simulink model "Ex5"  (R2024b)
settings: Solver=VariableStepAuto  StartTime=0.0  StopTime=100  RelTol=1e-3
settings Model: Creator=eduardo  LastModifiedBy=eduardo
settings DataIOCC: SaveFormat=Array  ReturnWorkspaceOutputs=off

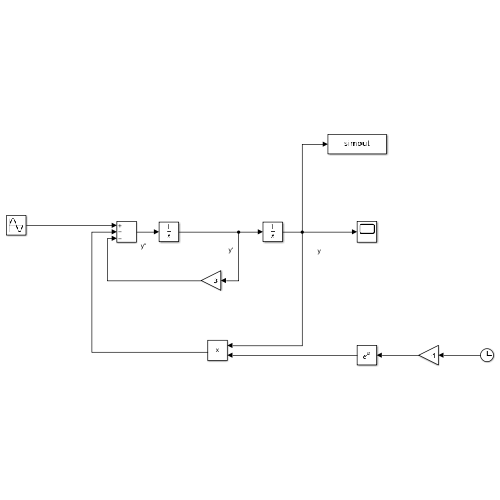
[thumbnail: Simulink's stored preview of the top-level diagram]
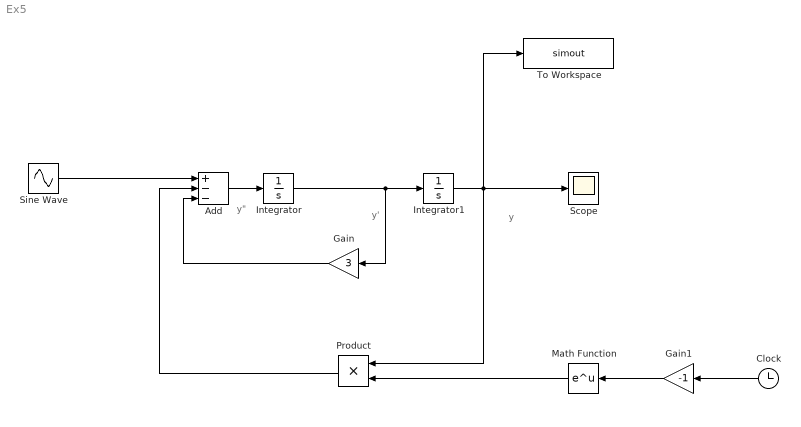
== system Ex5 ==
  note: y
  note: y'
  note: y"
  Add : Sum  Inputs=+--
  Clock : Clock
  Gain : Gain  Gain=3
  Gain1 : Gain  Gain=-1
  Integrator : Integrator
  Integrator1 : Integrator
  Math Function : Math
  Product : Product
  Scope : Scope
  Sine Wave : Sin  Amplitude=8  Frequency=5  SampleTime=0
  To Workspace : ToWorkspace  VariableName=simout  SampleTime=-1
  wires:
  Integrator/1 -> Gain/1, Integrator1/1
  Integrator1/1 -> To Workspace/1, Product/1, Scope/1
  Add/1 -> Integrator/1
  Gain/1 -> Add/3
  Sine Wave/1 -> Add/1
  Product/1 -> Add/2
  Math Function/1 -> Product/2
  Gain1/1 -> Math Function/1
  Clock/1 -> Gain1/1
